simulink model "simulate_fixed_plus_quad"  (R2021a)
settings: Solver=VariableStepAuto  StartTime=0.0  StopTime=600  RelTol=1e-3
PreLoadFcn:
  | set_param_fixed_complex;
undefined symbols (not defined in the file or in its folder): ParamFixComplex, ParamQuad
settings Model: PacingRate=1000  Creator=diogo  LastModifiedBy=Nunes
settings SolverCC: AlgebraicLoopSolver=TrustRegion
settings DebuggingCC: SFMachineParentedDataDiag=warning

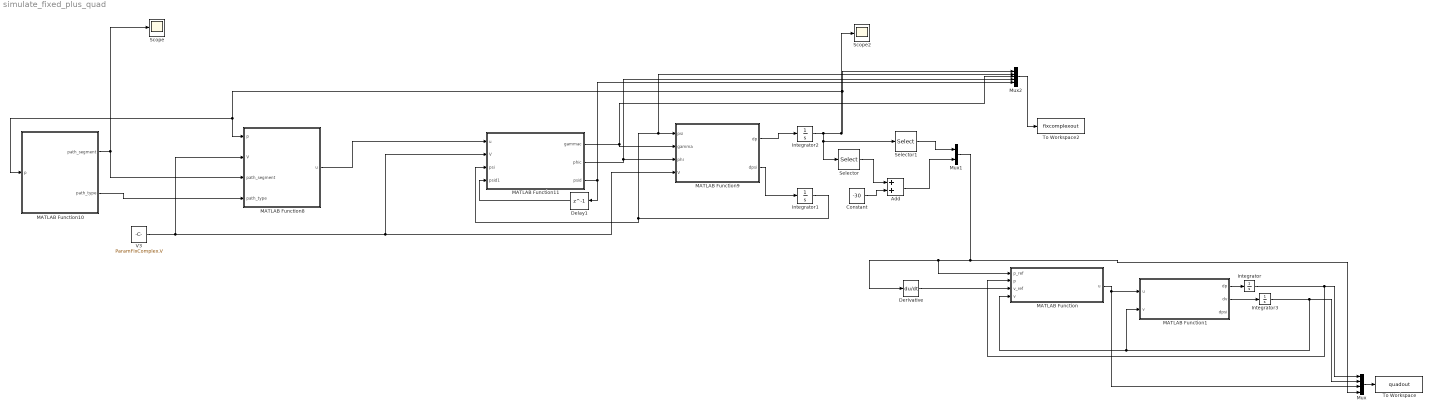
== system simulate_fixed_plus_quad ==
  Add : Sum
  Constant : Constant  Value=-30
  Delay1 : Delay  DelayLength=1  InitialCondition=0
  Derivative : Derivative
  Integrator : Integrator  InitialCondition=ParamQuad.p0
  Integrator1 : Integrator  InitialCondition=ParamFixComplex.psi0
  Integrator2 : Integrator  InitialCondition=ParamFixComplex.p0
  Integrator3 : Integrator  InitialCondition=ParamQuad.v0
  MATLAB Function : MATLAB Function  TreatAsAtomicUnit=on
  MATLAB Function1 : MATLAB Function  TreatAsAtomicUnit=on
  MATLAB Function10 : MATLAB Function  TreatAsAtomicUnit=on
  MATLAB Function11 : MATLAB Function  TreatAsAtomicUnit=on
  MATLAB Function8 : MATLAB Function  TreatAsAtomicUnit=on
  MATLAB Function9 : MATLAB Function  TreatAsAtomicUnit=on
  Mux : Mux
  Mux1 : Mux  Inputs=2
  Mux2 : Mux  Inputs=5
  Scope : Scope
  Scope2 : Scope
  Selector : Selector  InputPortWidth=3  IndexOptions=Index vector (dialog)  Indices=[ 3]  OutputSizes=1
  Selector1 : Selector  InputPortWidth=3  IndexOptions=Index vector (dialog)  Indices=[ 1 2]  OutputSizes=1
  To Workspace : ToWorkspace  VariableName=quadout  SaveFormat=Timeseries  SampleTime=-1
  To Workspace2 : ToWorkspace  VariableName=fixcomplexout  SaveFormat=Timeseries  SampleTime=-1
  V3 : Constant  Value=ParamFixComplex.V
  wires:
  MATLAB Function11/3(psid) -> Mux2/5, Delay1/1
  Delay1/1 -> MATLAB Function11/4(psid1)
  V3/1 -> MATLAB Function8/2(V), MATLAB Function11/2(V), MATLAB Function9/4(V)
  MATLAB Function11/1(gammac) -> Mux2/3, MATLAB Function9/2(gamma)
  Mux2/1 -> To Workspace2/1
  MATLAB Function8/1(u) -> MATLAB Function11/1(u)
  MATLAB Function9/1(dp) -> Integrator2/1
  MATLAB Function9/2(dpsi) -> Integrator1/1
  MATLAB Function11/2(phic) -> Mux2/4, MATLAB Function9/3(phi)
  Integrator1/1 -> MATLAB Function11/3(psi), Mux2/2, MATLAB Function9/1(psi)
  MATLAB Function10/1(path_segment) -> Scope/1, MATLAB Function8/3(path_segment)
  MATLAB Function10/2(path_type) -> MATLAB Function8/4(path_type)
  Derivative/1 -> MATLAB Function/3(v_ref)
  Integrator3/1 -> Mux/2, MATLAB Function/4(v), MATLAB Function1/2(v)
  MATLAB Function/1(u) -> MATLAB Function1/1(u), Mux/3
  MATLAB Function1/1(dp) -> Integrator/1
  Integrator/1 -> Mux/1, MATLAB Function/2(p)
  Integrator2/1 -> Selector1/1, Selector/1, Mux2/1, MATLAB Function8/1(p), MATLAB Function10/1(p), Scope2/1
  MATLAB Function1/2(dv) -> Integrator3/1
  Mux/1 -> To Workspace/1
  Mux1/1 -> Derivative/1, MATLAB Function/1(p_ref), Mux/4
  Constant/1 -> Add/2
  Selector/1 -> Add/1
  Add/1 -> Mux1/2
  Selector1/1 -> Mux1/1

== matlab function simulate_fixed_plus_quad/MATLAB Function1 ==
  data: u input; v input; dp output; dv output; ParamQuad parameter; dpsi output
function [dp,dv,dpsi] = drone_model(u,v,ParamQuad)
%DRONE_MODEL Summary of this function goes here
%   Detailed explanation goes here

 
    
    dp = v;
    dv = [0;0;9.8] + 1/ParamQuad.m*u;
    dpsi = 0;
    
end

== matlab function simulate_fixed_plus_quad/MATLAB Function ==
  data: p_ref input; p input; v_ref input; u output; v input; ParamQuad parameter
function u = drone_controller(p_ref,p,v_ref,v,ParamQuad)
%DRONE_CONTROLLER Summary of this function goes here
%   Detailed explanation goes here

  
    
    u = -diag([ParamQuad.kp/2,ParamQuad.kp/2,ParamQuad.kp])*(p-p_ref) + ...
        -diag([ParamQuad.kv/2,ParamQuad.kv/2,ParamQuad.kv])*(v-v_ref) - [0;0;ParamQuad.m*9.8];
    
end

== matlab function simulate_fixed_plus_quad/MATLAB Function8 ==
  settings: updateMethod=DISCRETE  sampleTime=ParamFixComplex.Ts
  data: p input; u output size=3; V input; ParamFixComplex parameter; path_segment input; path_type input
function u  = complex_path_generator(p, V, ParamFixComplex, path_segment, path_type)



if path_type == 0                %straight line following
    %Variables

    psi_l = ParamFixComplex.psi_l(path_segment);  %desired heading angle
    gamma_l = ParamFixComplex.gamma_l(path_segment); %desired flight path angle

    c_n = ParamFixComplex.c0(1,path_segment);    %path starting point
    c_e = ParamFixComplex.c0(2,path_segment);
    c_d = ParamFixComplex.c0(3,path_segment);
    
    
    r_n = p(1);    %position
    r_e = p(2);
    r_d = p(3);
    r = [r_n; r_e; r_d];

    cl = [c_n; c_e; c_d];

    n_lon = [ -sin(psi_l) ; cos(psi_l) ; 0 ]; 

    n_lat = [-cos(psi_l)*sin(gamma_l) ; -sin(psi_l)*sin(gamma_l) ; -cos(gamma_l) ];

     k1 = ParamFixComplex.k1_line;
    k2 = ParamFixComplex.k2_line;


    %u_line = k1*(n_lon*transpose(n_lon) +  n_lat*transpose(n_lat))*(r - cl) + k2*cross(n_lon,n_lat);
    u_line = -k1*(n_lon*n_lon' +  n_lat*n_lat')*(r - cl) - k2*cross(n_lon,n_lat);

    u = V*(u_line/norm(u_line));

% if  any(isnan(n_lon)) || any(isnan(n_lat))
%     xpto = 0;
% end
    
else                            %orbit following  
    %Variables

     Rh = ParamFixComplex.Rh(path_segment);
     lambda = ParamFixComplex.lambda(path_segment);
     gamma_h = ParamFixComplex.gamma_h(path_segment);
     psi_h = ParamFixComplex.psi_h(path_segment);

    k1 = ParamFixComplex.k1_orb;
    k2 = ParamFixComplex.k2_orb;



    c_n = ParamFixComplex.c0(1,path_segment);   %center of helix
    c_e = ParamFixComplex.c0(2,path_segment);
    c_d = ParamFixComplex.c0(3,path_segment);

     r_n = p(1);
     r_e = p(2);
     r_d = p(3);




    dalpha_cyl =  [ 2*(r_n - c_n)/Rh ; 2*(r_e - c_e)/Rh ; 0 ] ;

    dalpha_pl = [ (tan(gamma_h)/lambda)*(-(r_e - c_e))/( (r_n - c_n)^2 + (r_e - c_e)^2 ) ; (tan(gamma_h)/lambda)*(r_n - c_n)/( (r_n - c_n)^2 + (r_e - c_e)^2 )  ; 1/Rh ] ;


    alpha_cyl = ( (r_n - c_n)/Rh )^2 + ( (r_e - c_e)/Rh )^2 -1;

    alpha_pl = ( (r_d - c_d)/Rh )^2 + (tan(gamma_h)/lambda)*(atan( (r_e - c_e)/(r_n - c_n) ) - psi_h);

    u_line = k1*(-alpha_cyl*dalpha_cyl + alpha_pl*dalpha_pl) - lambda*k2*( (2/Rh)*[ (r_e - c_e)/Rh ; -(r_n - c_n)/Rh ; lambda*tan(gamma_h) ]) ;

    u =  V*(u_line/norm(u_line));

% if  any(isnan(dalpha_cyl)) || any(isnan(dalpha_pl))
%     xpto = 0;
% end

end




% if any(isnan(u)) || any(isnan(u_line)) 
%     xpto = 0;
% end


end

== matlab function simulate_fixed_plus_quad/MATLAB Function9 ==
  data: psi input; gamma input; phi input; V input; dp output; dpsi output
function [dp,dpsi] = drone_model(psi,gamma,phi, V)
    
    %criar param para generalizar os valores
    
    %dp = [V*cos(psi)*cos(gamma); V*sin(psi)*cos(gamma); -V*sin(gamma)]
    
    dpn =V*cos(psi)*cos(gamma);
    dpe = V*sin(psi)*cos(gamma);
    dpd = -V*sin(gamma);
    dpsi =  (9.8/V)*tan(phi);
    
    dp = [dpn; dpe; dpd];
    if any(isnan(dp))
    xpto = 0;
    end
end

== matlab function simulate_fixed_plus_quad/MATLAB Function10 ==
  settings: updateMethod=DISCRETE  sampleTime=ParamFixComplex.Ts
  data: p input; path_segment output; ParamFixComplex parameter; path_type output
function [path_segment, path_type]  = complex_path_manager(p,  ParamFixComplex)

persistent path_segment2;
if isempty(path_segment2)
        path_segment2 = 1;
end

path_segment = path_segment2;

number_of_segments = size(ParamFixComplex.paths);
number_of_segments = number_of_segments(2);



proximity_radius = ParamFixComplex.proximity_to_next_path ;

if ~(path_segment == number_of_segments)
         
   % c_n = ParamFixComplex.c0(1, path_segment );    
   % c_e = ParamFixComplex.c0(2,path_segment );
   % c_d = ParamFixComplex.c0(3,path_segment); 
%else 
    
    c_n = ParamFixComplex.c0(1, path_segment + 1);   
    c_e = ParamFixComplex.c0(2,path_segment + 1);
    c_d = ParamFixComplex.c0(3,path_segment + 1);
    
    path_type_next = ParamFixComplex.paths(path_segment + 1);
    
    distance_to_next_path = sqrt((c_n - p(1))^2 + (c_e - p(2))^2 + (c_d - p(3))^2);


    if path_type_next == 0
        if distance_to_next_path < proximity_radius
            path_segment = path_segment + 1 ;

        end
    else
        if distance_to_next_path < (proximity_radius + ParamFixComplex.Rh(path_segment + 1))  %if it's close to any point from the inside of the helix
            path_segment = path_segment + 1 ;
        end
    end

    

end




path_segment2 = path_segment;
path_type = ParamFixComplex.paths(path_segment);



end


















% if distance_to_next_path < proximity_radius
%     segment = 2;

% %second line starting point
% c_n = ParamFixComplex.c0_l(1, segmentPrevious + 1);   
% c_e = ParamFixComplex.c0_l(2,segmentPrevious + 1);
% c_d = ParamFixComplex.c0_l(3,segmentPrevious + 1);
% 
% 
% distance_to_next_path = sqrt((c_n - p(1))^2 + (c_e - p(2))^2 + (c_d - p(3))^2);
% proximity_radius = 10;
% 
% 
% if distance_to_next_path < proximity_radius
%     segment = 2;
% 
% else 
%     segment = segmentPrevious;
% end
% 
% % path_segment = segment;

== matlab function simulate_fixed_plus_quad/MATLAB Function11 ==
  settings: updateMethod=DISCRETE  sampleTime=ParamFixComplex.Ts
  data: u input; V input; psi input; psid1 input; gammac output; phic output; ParamFixComplex parameter; psid output
function [  gammac, phic, psid] = path_following_controller(u, V, psi, psid1, ParamFixComplex)

gamma_limit = ParamFixComplex.gamma_limit;
phi_limit = ParamFixComplex.phi_limit;
kphi = ParamFixComplex.kphi;

gammac = -sat(asin(u(3,1)/V), gamma_limit);

psid = atan2(u(2,1),u(1,1));

while abs(psid - psid1) > 3*pi/2
    if((psid - psid1) > 3*pi/2) 
        psid = psid- 2*pi;
    elseif ((psid - psid1) < - 3*pi/2)
        psid = psid + 2*pi;
    end
end

%if(abs(psid - psid1) > pi)
%    xpto = 0;
%end;

phic = sat(kphi*(psid - psi), phi_limit);

% if isnan(gammac) || isnan(phic)
%     xpto = 0;
% end
%     

end
